simulink model "FDM"  (R2021b)
settings: Solver=ode4  StartTime=0.0  StopTime=15  FixedStep=0.02  RelTol=1e-3
values from neighbouring files (symbols this model uses):
  k = 0.04    [Aircraft.m]
  m = 100000    [Aircraft.m]    (also in BFZ100.mat = 10)
undefined symbols (not defined in the file or in its folder): d
settings Model: Creator=jonih  LastModifiedBy=jonih

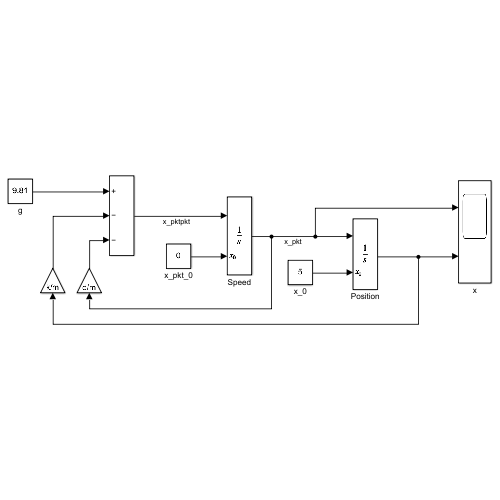
[thumbnail: Simulink's stored preview of the top-level diagram]
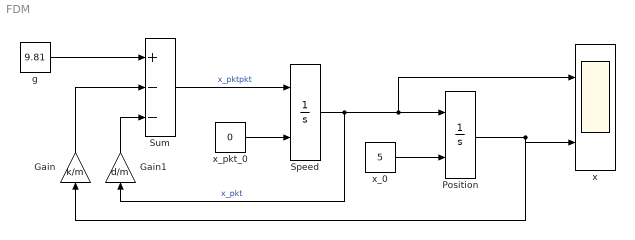
== system FDM ==
  Gain : Gain  Gain=k/m
  Gain1 : Gain  Gain=d/m
  Position : Integrator  InitialConditionSource=external  ContinuousStateAttributes='Position'
  Speed : Integrator  InitialConditionSource=external  ContinuousStateAttributes='speed'
  Sum : Sum  Inputs=+--
  g : Constant  Value=9.81
  x : Scope  NumInputPorts=2
  x_0 : Constant  Value=5
  x_pkt_0 : Constant  Value=0
  wires:
  Speed/1 -> Gain1/1, x/1, Position/1  "x_pkt"
  Sum/1 -> Speed/1  "x_pktpkt"
  x_pkt_0/1 -> Speed/2
  x_0/1 -> Position/2
  Position/1 -> x/2, Gain/1
  Gain/1 -> Sum/2
  Gain1/1 -> Sum/3
  g/1 -> Sum/1
